simulink model "case2"  (R2024b)
settings: Solver=FixedStepAuto  StartTime=0  StopTime=1  FixedStep=1e-7  RelTol=1e-3
values from neighbouring files (symbols this model uses):
  SG_D_1_D = 0.01056    [IEEE9_case_parameters.m]    (also in case1_parameters.m; case2_parameters.m; case3_parameters.m; case4_parameters.m)
  SG_D_1_EnableSaturation = 0    [IEEE9_case_parameters.m]    (also in case1_parameters.m; case2_parameters.m; case3_parameters.m; case4_parameters.m)
  SG_D_1_f0 = 60    [IEEE9_case_parameters.m]    (also in case1_parameters.m; case2_parameters.m; case3_parameters.m; case4_parameters.m)
  SG_D_1_H = 7.5    [IEEE9_case_parameters.m]    (also in case1_parameters.m; case2_parameters.m; case3_parameters.m; case4_parameters.m)
  SG_D_1_K_A = 20    [IEEE9_case_parameters.m]    (also in case1_parameters.m; case2_parameters.m; case3_parameters.m; case4_parameters.m)
  SG_D_1_K_E = 1.000000e+1    (= 10)    [IEEE9_case_parameters.m]    (also in case1_parameters.m; case2_parameters.m; case3_parameters.m; case4_parameters.m)
  SG_D_1_K_F = 2.363    [IEEE9_case_parameters.m]    (also in case1_parameters.m; case2_parameters.m; case3_parameters.m; case4_parameters.m)
  SG_D_1_K_s = 0.5    [IEEE9_case_parameters.m]    (also in case1_parameters.m = 5; case2_parameters.m = 5; case3_parameters.m = 5; case4_parameters.m = 5)
  SG_D_1_R_a = 0.001088    [IEEE9_case_parameters.m]    (also in case1_parameters.m; case2_parameters.m; case3_parameters.m; case4_parameters.m)
  SG_D_1_S_A = 1    [IEEE9_case_parameters.m]    (also in case1_parameters.m; case2_parameters.m; case3_parameters.m; case4_parameters.m)
  SG_D_1_S_B = 0.103    [IEEE9_case_parameters.m]    (also in case1_parameters.m; case2_parameters.m; case3_parameters.m; case4_parameters.m)
  SG_D_1_S_N = 10.659857    [IEEE9_case_parameters.m]    (also in case1_parameters.m; case2_parameters.m; case3_parameters.m; case4_parameters.m)
  SG_D_1_SpeedPara = 200    [IEEE9_case_parameters.m]    (also in case1_parameters.m; case2_parameters.m; case3_parameters.m; case4_parameters.m)
  SG_D_1_T_0 = 0.720173    [IEEE9_case_parameters.m]    (also in case1_parameters.m = 0.755522; case2_parameters.m = 0.808931; case3_parameters.m = 0.869402; case4_parameters.m = 0.729316)
  SG_D_1_T_1 = 0.3    [IEEE9_case_parameters.m]    (also in case1_parameters.m; case2_parameters.m; case3_parameters.m; case4_parameters.m)
  SG_D_1_T_2 = 0.05    [IEEE9_case_parameters.m]    (also in case1_parameters.m; case2_parameters.m; case3_parameters.m; case4_parameters.m)
  SG_D_1_T_3 = 0.02    [IEEE9_case_parameters.m]    (also in case1_parameters.m; case2_parameters.m; case3_parameters.m; case4_parameters.m)
  SG_D_1_T_4 = 0.005    [IEEE9_case_parameters.m]    (also in case1_parameters.m; case2_parameters.m; case3_parameters.m; case4_parameters.m)
  SG_D_1_T_A = 0.02    [IEEE9_case_parameters.m]    (also in case1_parameters.m; case2_parameters.m; case3_parameters.m; case4_parameters.m)
  SG_D_1_T_dd = 8.000000e+0    (= 8)    [IEEE9_case_parameters.m]    (also in case1_parameters.m; case2_parameters.m; case3_parameters.m; case4_parameters.m)
  SG_D_1_T_ddd = 0.04    [IEEE9_case_parameters.m]    (also in case1_parameters.m; case2_parameters.m; case3_parameters.m; case4_parameters.m)
  SG_D_1_T_E = 0.314    [IEEE9_case_parameters.m]    (also in case1_parameters.m; case2_parameters.m; case3_parameters.m; case4_parameters.m)
  SG_D_1_T_F = 0.35    [IEEE9_case_parameters.m]    (also in case1_parameters.m; case2_parameters.m; case3_parameters.m; case4_parameters.m)
  SG_D_1_T_qd = 0.8    [IEEE9_case_parameters.m]    (also in case1_parameters.m; case2_parameters.m; case3_parameters.m; case4_parameters.m)
  SG_D_1_T_qdd = 0.02    [IEEE9_case_parameters.m]    (also in case1_parameters.m; case2_parameters.m; case3_parameters.m; case4_parameters.m)
  SG_D_1_T_speed = 0.1    [IEEE9_case_parameters.m]    (also in case1_parameters.m = 200; case2_parameters.m = 200; case3_parameters.m = 200; case4_parameters.m = 200)
  SG_D_1_T_w = 0.5    [IEEE9_case_parameters.m]    (also in case1_parameters.m; case2_parameters.m; case3_parameters.m; case4_parameters.m)
  SG_D_1_V_ref = 1.990276    [IEEE9_case_parameters.m]    (also in case1_parameters.m = 2.042296; case2_parameters.m = 2.051388; case3_parameters.m = 2.089584; case4_parameters.m = 2.01845)
  SG_D_1_w_ref = 376.991118    [IEEE9_case_parameters.m]    (also in case1_parameters.m; case2_parameters.m; case3_parameters.m; case4_parameters.m)
  SG_D_1_wb = 6.000000e+1    (= 60)    [IEEE9_case_parameters.m]    (also in case1_parameters.m; case2_parameters.m; case3_parameters.m; case4_parameters.m)
  SG_D_1_x_d = 1.9    [IEEE9_case_parameters.m]    (also in case1_parameters.m; case2_parameters.m; case3_parameters.m; case4_parameters.m)
  SG_D_1_x_dd = 0.302    [IEEE9_case_parameters.m]    (also in case1_parameters.m; case2_parameters.m; case3_parameters.m; case4_parameters.m)
  SG_D_1_x_ddd = 0.204    [IEEE9_case_parameters.m]    (also in case1_parameters.m; case2_parameters.m; case3_parameters.m; case4_parameters.m)
  SG_D_1_x_l = 0.05    [IEEE9_case_parameters.m]    (also in case1_parameters.m; case2_parameters.m; case3_parameters.m; case4_parameters.m)
  SG_D_1_x_q = 1.3    [IEEE9_case_parameters.m]    (also in case1_parameters.m; case2_parameters.m; case3_parameters.m; case4_parameters.m)
  SG_D_1_x_qd = 0.5    [IEEE9_case_parameters.m]    (also in case1_parameters.m; case2_parameters.m; case3_parameters.m; case4_parameters.m)
  SG_D_1_x_qdd = 0.3    [IEEE9_case_parameters.m]    (also in case1_parameters.m; case2_parameters.m; case3_parameters.m; case4_parameters.m)
  SG_D_2_D = 0.02    [IEEE9_case_parameters.m]    (also in case1_parameters.m; case2_parameters.m; case3_parameters.m; case4_parameters.m)
  SG_D_2_EnableSaturation = 0    [IEEE9_case_parameters.m]    (also in case1_parameters.m; case2_parameters.m; case3_parameters.m; case4_parameters.m)
  SG_D_2_f0 = 60    [IEEE9_case_parameters.m]    (also in case1_parameters.m; case2_parameters.m; case3_parameters.m; case4_parameters.m)
  SG_D_2_H = 8.000000e+0    (= 8)    [IEEE9_case_parameters.m]    (also in case1_parameters.m; case2_parameters.m; case3_parameters.m; case4_parameters.m)
  SG_D_2_K_A = 20    [IEEE9_case_parameters.m]    (also in case1_parameters.m; case2_parameters.m; case3_parameters.m; case4_parameters.m)
  SG_D_2_K_E = 1.000000e+1    (= 10)    [IEEE9_case_parameters.m]    (also in case1_parameters.m; case2_parameters.m; case3_parameters.m; case4_parameters.m)
  SG_D_2_K_F = 2.363    [IEEE9_case_parameters.m]    (also in case1_parameters.m; case2_parameters.m; case3_parameters.m; case4_parameters.m)
  SG_D_2_K_s = 0.5    [IEEE9_case_parameters.m]    (also in case1_parameters.m = 4; case2_parameters.m = 4; case3_parameters.m = 4; case4_parameters.m = 4)
  SG_D_2_R_a = 0.001088    [IEEE9_case_parameters.m]    (also in case1_parameters.m; case2_parameters.m; case3_parameters.m; case4_parameters.m)
  SG_D_2_S_A = 1    [IEEE9_case_parameters.m]    (also in case1_parameters.m; case2_parameters.m; case3_parameters.m; case4_parameters.m)
  SG_D_2_S_B = 0.103    [IEEE9_case_parameters.m]    (also in case1_parameters.m; case2_parameters.m; case3_parameters.m; case4_parameters.m)
  SG_D_2_S_N = 10.659857    [IEEE9_case_parameters.m]    (also in case1_parameters.m; case2_parameters.m; case3_parameters.m; case4_parameters.m)
  SG_D_2_SpeedPara = 200    [IEEE9_case_parameters.m]    (also in case1_parameters.m; case2_parameters.m; case3_parameters.m; case4_parameters.m)
  SG_D_2_T_0 = 1.632913    [IEEE9_case_parameters.m]    (also in case1_parameters.m = 1.632925; case2_parameters.m = 1.632915; case3_parameters.m = 1.632914; case4_parameters.m = 1.632927)
  SG_D_2_T_1 = 0.2    [IEEE9_case_parameters.m]    (also in case1_parameters.m; case2_parameters.m; case3_parameters.m; case4_parameters.m)
  SG_D_2_T_2 = 0.05    [IEEE9_case_parameters.m]    (also in case1_parameters.m; case2_parameters.m; case3_parameters.m; case4_parameters.m)
  SG_D_2_T_3 = 0.02    [IEEE9_case_parameters.m]    (also in case1_parameters.m; case2_parameters.m; case3_parameters.m; case4_parameters.m)
  SG_D_2_T_4 = 0.005    [IEEE9_case_parameters.m]    (also in case1_parameters.m; case2_parameters.m; case3_parameters.m; case4_parameters.m)
  SG_D_2_T_A = 0.02    [IEEE9_case_parameters.m]    (also in case1_parameters.m; case2_parameters.m; case3_parameters.m; case4_parameters.m)
  SG_D_2_T_dd = 7.9    [IEEE9_case_parameters.m]    (also in case1_parameters.m; case2_parameters.m; case3_parameters.m; case4_parameters.m)
  SG_D_2_T_ddd = 0.04    [IEEE9_case_parameters.m]    (also in case1_parameters.m; case2_parameters.m; case3_parameters.m; case4_parameters.m)
  SG_D_2_T_E = 0.314    [IEEE9_case_parameters.m]    (also in case1_parameters.m; case2_parameters.m; case3_parameters.m; case4_parameters.m)
  SG_D_2_T_F = 0.35    [IEEE9_case_parameters.m]    (also in case1_parameters.m; case2_parameters.m; case3_parameters.m; case4_parameters.m)
  SG_D_2_T_qd = 0.8    [IEEE9_case_parameters.m]    (also in case1_parameters.m; case2_parameters.m; case3_parameters.m; case4_parameters.m)
  SG_D_2_T_qdd = 0.015    [IEEE9_case_parameters.m]    (also in case1_parameters.m; case2_parameters.m; case3_parameters.m; case4_parameters.m)
  SG_D_2_T_speed = 0.1    [IEEE9_case_parameters.m]    (also in case1_parameters.m = 150; case2_parameters.m = 150; case3_parameters.m = 150; case4_parameters.m = 150)
  SG_D_2_T_w = 0.35    [IEEE9_case_parameters.m]    (also in case1_parameters.m; case2_parameters.m; case3_parameters.m; case4_parameters.m)
  SG_D_2_V_ref = 2.58547    [IEEE9_case_parameters.m]    (also in case1_parameters.m = 2.597896; case2_parameters.m = 2.587136; case3_parameters.m = 2.586042; case4_parameters.m = 2.599679)
  SG_D_2_w_ref = 376.991118    [IEEE9_case_parameters.m]    (also in case1_parameters.m; case2_parameters.m; case3_parameters.m; case4_parameters.m)
  SG_D_2_wb = 6.000000e+1    (= 60)    [IEEE9_case_parameters.m]    (also in case1_parameters.m; case2_parameters.m; case3_parameters.m; case4_parameters.m)
  SG_D_2_x_d = 1.8    [IEEE9_case_parameters.m]    (also in case1_parameters.m; case2_parameters.m; case3_parameters.m; case4_parameters.m)
  SG_D_2_x_dd = 0.302    [IEEE9_case_parameters.m]    (also in case1_parameters.m; case2_parameters.m; case3_parameters.m; case4_parameters.m)
  SG_D_2_x_ddd = 0.204    [IEEE9_case_parameters.m]    (also in case1_parameters.m; case2_parameters.m; case3_parameters.m; case4_parameters.m)
  SG_D_2_x_l = 0.05    [IEEE9_case_parameters.m]    (also in case1_parameters.m; case2_parameters.m; case3_parameters.m; case4_parameters.m)
  SG_D_2_x_q = 1.25    [IEEE9_case_parameters.m]    (also in case1_parameters.m; case2_parameters.m; case3_parameters.m; case4_parameters.m)
  SG_D_2_x_qd = 0.5    [IEEE9_case_parameters.m]    (also in case1_parameters.m; case2_parameters.m; case3_parameters.m; case4_parameters.m)
  SG_D_2_x_qdd = 0.3    [IEEE9_case_parameters.m]    (also in case1_parameters.m; case2_parameters.m; case3_parameters.m; case4_parameters.m)
  SG_D_3_D = 0.02    [IEEE9_case_parameters.m]    (also in case1_parameters.m; case2_parameters.m; case3_parameters.m; case4_parameters.m)
  SG_D_3_EnableSaturation = 0    [IEEE9_case_parameters.m]    (also in case1_parameters.m; case2_parameters.m; case3_parameters.m; case4_parameters.m)
  SG_D_3_f0 = 60    [IEEE9_case_parameters.m]    (also in case1_parameters.m; case2_parameters.m; case3_parameters.m; case4_parameters.m)
  SG_D_3_H = 7.7    [IEEE9_case_parameters.m]    (also in case1_parameters.m; case2_parameters.m; case3_parameters.m; case4_parameters.m)
  SG_D_3_K_A = 20    [IEEE9_case_parameters.m]    (also in case1_parameters.m; case2_parameters.m; case3_parameters.m; case4_parameters.m)
  SG_D_3_K_E = 1.000000e+1    (= 10)    [IEEE9_case_parameters.m]    (also in case1_parameters.m; case2_parameters.m; case3_parameters.m; case4_parameters.m)
  SG_D_3_K_F = 2.363    [IEEE9_case_parameters.m]    (also in case1_parameters.m; case2_parameters.m; case3_parameters.m; case4_parameters.m)
  SG_D_3_K_s = 0.2    [IEEE9_case_parameters.m]    (also in case1_parameters.m = 2; case2_parameters.m = 2; case3_parameters.m = 2; case4_parameters.m = 2)
  SG_D_3_R_a = 0.001088    [IEEE9_case_parameters.m]    (also in case1_parameters.m; case2_parameters.m; case3_parameters.m; case4_parameters.m)
  SG_D_3_S_A = 1    [IEEE9_case_parameters.m]    (also in case1_parameters.m; case2_parameters.m; case3_parameters.m; case4_parameters.m)
  SG_D_3_S_B = 0.103    [IEEE9_case_parameters.m]    (also in case1_parameters.m; case2_parameters.m; case3_parameters.m; case4_parameters.m)
  SG_D_3_S_N = 10.659857    [IEEE9_case_parameters.m]    (also in case1_parameters.m; case2_parameters.m; case3_parameters.m; case4_parameters.m)
  SG_D_3_SpeedPara = 200    [IEEE9_case_parameters.m]    (also in case1_parameters.m; case2_parameters.m; case3_parameters.m; case4_parameters.m)
  SG_D_3_T_0 = 0.850788    [IEEE9_case_parameters.m]    (also in case1_parameters.m = 0.850786; case2_parameters.m = 0.850787; case3_parameters.m; case4_parameters.m = 0.850786)
  SG_D_3_T_1 = 0.2    [IEEE9_case_parameters.m]    (also in case1_parameters.m; case2_parameters.m; case3_parameters.m; case4_parameters.m)
  SG_D_3_T_2 = 0.05    [IEEE9_case_parameters.m]    (also in case1_parameters.m; case2_parameters.m; case3_parameters.m; case4_parameters.m)
  SG_D_3_T_3 = 0.02    [IEEE9_case_parameters.m]    (also in case1_parameters.m; case2_parameters.m; case3_parameters.m; case4_parameters.m)
  SG_D_3_T_4 = 0.005    [IEEE9_case_parameters.m]    (also in case1_parameters.m; case2_parameters.m; case3_parameters.m; case4_parameters.m)
  SG_D_3_T_A = 0.02    [IEEE9_case_parameters.m]    (also in case1_parameters.m; case2_parameters.m; case3_parameters.m; case4_parameters.m)
  SG_D_3_T_dd = 8.1    [IEEE9_case_parameters.m]    (also in case1_parameters.m; case2_parameters.m; case3_parameters.m; case4_parameters.m)
  SG_D_3_T_ddd = 0.04    [IEEE9_case_parameters.m]    (also in case1_parameters.m; case2_parameters.m; case3_parameters.m; case4_parameters.m)
  SG_D_3_T_E = 0.314    [IEEE9_case_parameters.m]    (also in case1_parameters.m; case2_parameters.m; case3_parameters.m; case4_parameters.m)
  SG_D_3_T_F = 0.35    [IEEE9_case_parameters.m]    (also in case1_parameters.m; case2_parameters.m; case3_parameters.m; case4_parameters.m)
  SG_D_3_T_qd = 0.8    [IEEE9_case_parameters.m]    (also in case1_parameters.m; case2_parameters.m; case3_parameters.m; case4_parameters.m)
  SG_D_3_T_qdd = 0.015    [IEEE9_case_parameters.m]    (also in case1_parameters.m; case2_parameters.m; case3_parameters.m; case4_parameters.m)
  SG_D_3_T_speed = 0.1    [IEEE9_case_parameters.m]    (also in case1_parameters.m = 180; case2_parameters.m = 180; case3_parameters.m = 180; case4_parameters.m = 180)
  SG_D_3_T_w = 0.4    [IEEE9_case_parameters.m]    (also in case1_parameters.m; case2_parameters.m; case3_parameters.m; case4_parameters.m)
  SG_D_3_V_ref = 1.892727    [IEEE9_case_parameters.m]    (also in case1_parameters.m = 1.906439; case2_parameters.m = 1.895535; case3_parameters.m = 1.892105; case4_parameters.m = 1.906598)
  SG_D_3_w_ref = 376.991118    [IEEE9_case_parameters.m]    (also in case1_parameters.m; case2_parameters.m; case3_parameters.m; case4_parameters.m)
  SG_D_3_wb = 6.000000e+1    (= 60)    [IEEE9_case_parameters.m]    (also in case1_parameters.m; case2_parameters.m; case3_parameters.m; case4_parameters.m)
  SG_D_3_x_d = 1.85    [IEEE9_case_parameters.m]    (also in case1_parameters.m; case2_parameters.m; case3_parameters.m; case4_parameters.m)
  SG_D_3_x_dd = 0.302    [IEEE9_case_parameters.m]    (also in case1_parameters.m; case2_parameters.m; case3_parameters.m; case4_parameters.m)
  SG_D_3_x_ddd = 0.204    [IEEE9_case_parameters.m]    (also in case1_parameters.m; case2_parameters.m; case3_parameters.m; case4_parameters.m)
  SG_D_3_x_l = 0.05    [IEEE9_case_parameters.m]    (also in case1_parameters.m; case2_parameters.m; case3_parameters.m; case4_parameters.m)
  SG_D_3_x_q = 1.2    [IEEE9_case_parameters.m]    (also in case1_parameters.m; case2_parameters.m; case3_parameters.m; case4_parameters.m)
  SG_D_3_x_qd = 0.5    [IEEE9_case_parameters.m]    (also in case1_parameters.m; case2_parameters.m; case3_parameters.m; case4_parameters.m)
  SG_D_3_x_qdd = 0.3    [IEEE9_case_parameters.m]    (also in case1_parameters.m; case2_parameters.m; case3_parameters.m; case4_parameters.m)
(part 5 of 12)

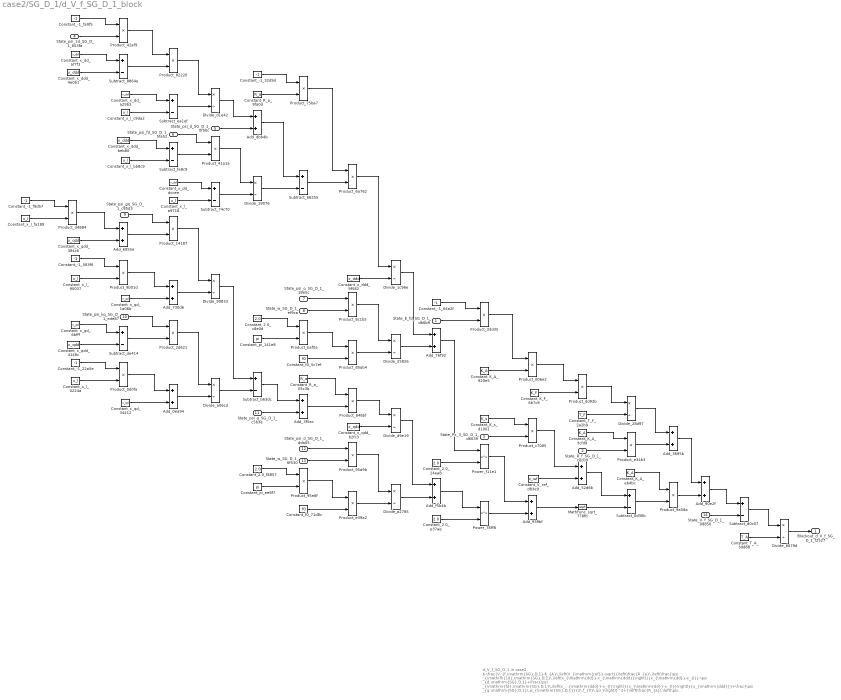
== system case2/SG_D_1/d_V_f_SG_D_1_block ==
  note: d_V_f_SG_D_1 in case2
      | $-\frac{V_{f,\mathrm{SG},D,1}-K_{A}\,\left(V_{\mathrm{ref}}-\sqrt{{\left(\frac{R_{a}\,\left(\frac{\psi _{\mathrm{1d},\mathrm{SG},D,1}\,\left(x_{\mathrm{dd}}-x_{\mathrm{ddd}}\right)}{x_{\mathrm{dd}}-x_{l}}-\psi _{d,\mathrm{SG},D,1}+\frac{\psi _{\mathrm{fd},\mathrm{SG},D,1}\,\left(x_{\mathrm{ddd}}-x_{l}\right)}{x_{\mathrm{dd}}-x_{l}}\right)}{x_{\mathrm{ddd}}}+\frac{\psi _{q,\mathrm{SG},D,1}\,w_{\mathrm{SG},D,1}}{2\,f_{0}\,\pi }\right)}^2+{\left(\frac{R_{a}\,\left(\psi _{q,\mathrm{SG},D,1}+\frac{\psi _{\mathrm{gq},\mathrm{SG},D,1}\,\left(x_{l}-x_{\mathrm{qdd}}\right)}{x_{l}-x_{\mathrm{qd}}}+\frac{\psi _{\mathrm{kq},\mathrm{SG},D,1}\,\left(x_{\mathrm{qd}}-x_{\mathrm{qdd}}\right)}{x_{l}-x_{\mathrm{qd}}}\right)}{x_{\mathrm{qdd}}}+\frac{\psi _{d,\mathrm{SG},D,1}\,w_{\mathrm{SG},D,1}}{2\,f_{0}\,\pi }\right)}^2}+K_{s}\,\mathrm{Px}_{3,\mathrm{SG},D,1}\right)-K_{A}\,R_{f,\mathrm{SG},D,1}+\frac{E_{\mathrm{fd},\mathrm{SG},D,1}\,K_{A}\,K_{F}}{T_{F}}}{T_{A}}$
      | Automatically generated on 2025-10-31 18:53:39 .
  State_E_fd_SG_D_1_db6b9 : Inport
  State_R_f_SG_D_1_cec09 : Inport  Port=2
  State_Px_3_SG_D_1_d6039 : Inport  Port=3
  State_psi_1d_SG_D_1_653fa : Inport  Port=4
  State_psi_d_SG_D_1_0f50c : Inport  Port=5
  State_psi_fd_SG_D_1_5fa52 : Inport  Port=6
  State_psi_q_SG_D_1_18e5c : Inport  Port=7
  State_w_SG_D_1_ef9ca : Inport  Port=8
  State_psi_gq_SG_D_1_c85d3 : Inport  Port=9
  State_psi_kq_SG_D_1_ede87 : Inport  Port=10
  State_psi_q_SG_D_1_c5b3e : Inport  Port=11
  State_psi_d_SG_D_1_dda05 : Inport  Port=12
  State_w_SG_D_1_6f530 : Inport  Port=13
  State_V_f_SG_D_1_0d850 : Inport  Port=14
  Add_0ea94 : Sum
  Add_3695b : Sum
  Add_3f5ac : Sum
  Add_52d6b : Sum
  Add_6955e : Sum
  Add_730d6 : Sum
  Add_76f92 : Sum
  Add_90e2f : Sum
  Add_939bf : Sum
  Add_dbb4b : Sum
  Add_f5b4b : Sum
  Constant_-1_22a5e : Constant  Value=-1
  Constant_-1_32d9d : Constant  Value=-1
  Constant_-1_583f6 : Constant  Value=-1
  Constant_-1_64a2f : Constant  Value=-1
  Constant_-1_f9d57 : Constant  Value=-1
  Constant_-1_fa9f5 : Constant  Value=-1
  Constant_2.0_24ea8 : Constant  Value=2.0
  Constant_2.0_c8e0d : Constant  Value=2.0
  Constant_2.0_e37ae : Constant  Value=2.0
  Constant_2.0_f8857 : Constant  Value=2.0
  Constant_K_A_3cfd9 : Constant  Value=K_A
  Constant_K_A_920e5 : Constant  Value=K_A
  Constant_K_A_eb4bc : Constant  Value=K_A
  Constant_K_F_6b7c9 : Constant  Value=K_F
  Constant_K_s_d1001 : Constant  Value=K_s
  Constant_R_a_05c3b : Constant  Value=R_a
  Constant_R_a_9fa0d : Constant  Value=R_a
  Constant_T_A_3dd88 : Constant  Value=T_A
  Constant_T_F_2a2b9 : Constant  Value=T_F
  Constant_V_ref_d83e9 : Constant  Value=V_ref
  Constant_f0_5c7ef : Constant  Value=f0
  Constant_f0_71d8c : Constant  Value=f0
  Constant_pi_141e8 : Constant  Value=pi
  Constant_pi_ee8f7 : Constant  Value=pi
  Constant_x_dd_a29b3 : Constant  Value=x_dd
  Constant_x_dd_af7f3 : Constant  Value=x_dd
  Constant_x_dd_dccee : Constant  Value=x_dd
  Constant_x_ddd_4e0b1 : Constant  Value=x_ddd
  Constant_x_ddd_9f582 : Constant  Value=x_ddd
  Constant_x_ddd_beb80 : Constant  Value=x_ddd
  Constant_x_l_0224a : Constant  Value=x_l
  Constant_x_l_90037 : Constant  Value=x_l
  Constant_x_l_a9718 : Constant  Value=x_l
  Constant_x_l_bb8c9 : Constant  Value=x_l
  Constant_x_l_c9da2 : Constant  Value=x_l
  Constant_x_l_fa189 : Constant  Value=x_l
  Constant_x_qd_1a06b : Constant  Value=x_qd
  Constant_x_qd_34412 : Constant  Value=x_qd
  Constant_x_qd_6bfff : Constant  Value=x_qd
  Constant_x_qdd_384c6 : Constant  Value=x_qdd
  Constant_x_qdd_4148c : Constant  Value=x_qdd
  Constant_x_qdd_b2fc3 : Constant  Value=x_qdd
  Divide_19076 : Product  Inputs=*/
  Divide_1c96e : Product  Inputs=*/
  Divide_25826 : Product  Inputs=*/
  Divide_28d97 : Product  Inputs=*/
  Divide_6679d : Product  Inputs=*/
  Divide_90833 : Product  Inputs=*/
  Divide_a06cd : Product  Inputs=*/
  Divide_a2785 : Product  Inputs=*/
  Divide_d1e42 : Product  Inputs=*/
  Divide_d9e19 : Product  Inputs=*/
  MathFunc_sqrt_778fb : Sqrt
  Power_35ff8 : Math  Operator=pow
  Power_f11e1 : Math  Operator=pow
  Product_006e2 : Product
  Product_0d0fa : Product
  Product_14187 : Product
  Product_2d621 : Product
  Product_33d35 : Product
  Product_41a1a : Product
  Product_42af9 : Product
  Product_6a762 : Product
  Product_75ba7 : Product
  Product_82220 : Product
  Product_848bf : Product
  Product_85ab4 : Product
  Product_8c1b5 : Product
  Product_95a9b : Product
  Product_95e8f : Product
  Product_9a58a : Product
  Product_9b01d : Product
  Product_baf0a : Product
  Product_c7085 : Product
  Product_d4884 : Product
  Product_dd92b : Product
  Product_e34b3 : Product
  Product_e39a2 : Product
  Subtract_0d36b : Sum  Inputs=+-
  Subtract_66255 : Sum  Inputs=+-
  Subtract_74c70 : Sum  Inputs=+-
  Subtract_8864e : Sum  Inputs=+-
  Subtract_b63dc : Sum  Inputs=+-
  Subtract_d0c07 : Sum  Inputs=+-
  Subtract_de414 : Sum  Inputs=+-
  Subtract_ea1ef : Sum  Inputs=+-
  Subtract_fa8c9 : Sum  Inputs=+-
  Blockout_d_V_f_SG_D_1_f2527 : Outport
  wires:
  Constant_-1_22a5e/1 -> Product_0d0fa/1
  Constant_-1_f9d57/1 -> Product_d4884/1
  State_psi_d_SG_D_1_dda05/1 -> Product_95a9b/1
  Constant_x_qd_34412/1 -> Add_0ea94/2
  Constant_x_qdd_384c6/1 -> Add_6955e/2
  State_w_SG_D_1_6f530/1 -> Product_95a9b/2
  Constant_x_l_fa189/1 -> Product_d4884/2
  Subtract_66255/1 -> Product_6a762/2
  Constant_x_l_0224a/1 -> Product_0d0fa/2
  Constant_x_dd_af7f3/1 -> Subtract_8864e/1
  Constant_R_a_9fa0d/1 -> Product_75ba7/2
  Constant_-1_fa9f5/1 -> Product_42af9/1
  Divide_19076/1 -> Subtract_66255/2
  Constant_x_ddd_4e0b1/1 -> Subtract_8864e/2
  Add_0ea94/1 -> Divide_a06cd/2
  State_psi_1d_SG_D_1_653fa/1 -> Product_42af9/2
  Add_730d6/1 -> Divide_90833/2
  Subtract_de414/1 -> Product_2d621/2
  Product_dd92b/1 -> Divide_28d97/1
  Product_baf0a/1 -> Product_85ab4/1
  Product_d4884/1 -> Add_6955e/1
  Constant_-1_583f6/1 -> Product_9b01d/1
  Constant_x_l_90037/1 -> Product_9b01d/2
  Add_dbb4b/1 -> Subtract_66255/1
  Constant_2.0_f8857/1 -> Product_95e8f/1
  Constant_x_qd_6bfff/1 -> Subtract_de414/1
  Product_42af9/1 -> Product_82220/1
  Constant_pi_ee8f7/1 -> Product_95e8f/2
  Constant_x_qdd_4148c/1 -> Subtract_de414/2
  Subtract_8864e/1 -> Product_82220/2
  State_psi_q_SG_D_1_c5b3e/1 -> Add_3f5ac/2
  Constant_x_dd_a29b3/1 -> Subtract_ea1ef/1
  Constant_x_l_c9da2/1 -> Subtract_ea1ef/2
  Constant_x_ddd_beb80/1 -> Subtract_fa8c9/1
  Constant_x_l_bb8c9/1 -> Subtract_fa8c9/2
  State_psi_gq_SG_D_1_c85d3/1 -> Product_14187/1
  Add_6955e/1 -> Product_14187/2
  Product_9b01d/1 -> Add_730d6/1
  Constant_x_qd_1a06b/1 -> Add_730d6/2
  Divide_d1e42/1 -> Add_dbb4b/1
  Subtract_ea1ef/1 -> Divide_d1e42/2
  State_psi_kq_SG_D_1_ede87/1 -> Product_2d621/1
  Divide_6679d/1 -> Blockout_d_V_f_SG_D_1_f2527/1
  Product_0d0fa/1 -> Add_0ea94/1
  Product_82220/1 -> Divide_d1e42/1
  State_psi_fd_SG_D_1_5fa52/1 -> Product_41a1a/1
  State_w_SG_D_1_ef9ca/1 -> Product_8c1b5/2
  Subtract_fa8c9/1 -> Product_41a1a/2
  Constant_x_dd_dccee/1 -> Subtract_74c70/1
  Constant_x_l_a9718/1 -> Subtract_74c70/2
  Product_14187/1 -> Divide_90833/1
  Product_75ba7/1 -> Product_6a762/1
  Product_2d621/1 -> Divide_a06cd/1
  State_psi_d_SG_D_1_0f50c/1 -> Add_dbb4b/2
  Product_41a1a/1 -> Divide_19076/1
  Subtract_74c70/1 -> Divide_19076/2
  Divide_90833/1 -> Subtract_b63dc/1
  Divide_a06cd/1 -> Subtract_b63dc/2
  Constant_-1_32d9d/1 -> Product_75ba7/1
  Constant_2.0_c8e0d/1 -> Product_baf0a/1
  Constant_pi_141e8/1 -> Product_baf0a/2
  Subtract_b63dc/1 -> Add_3f5ac/1
  State_psi_q_SG_D_1_18e5c/1 -> Product_8c1b5/1
  Constant_f0_5c7ef/1 -> Product_85ab4/2
  Constant_R_a_05c3b/1 -> Product_848bf/1
  Add_3f5ac/1 -> Product_848bf/2
  Product_95e8f/1 -> Product_e39a2/1
  Power_f11e1/1 -> Add_939bf/1
  Constant_f0_71d8c/1 -> Product_e39a2/2
  Product_6a762/1 -> Divide_1c96e/1
  Constant_x_ddd_9f582/1 -> Divide_1c96e/2
  Product_8c1b5/1 -> Divide_25826/1
  Product_85ab4/1 -> Divide_25826/2
  Product_848bf/1 -> Divide_d9e19/1
  Constant_x_qdd_b2fc3/1 -> Divide_d9e19/2
  Product_95a9b/1 -> Divide_a2785/1
  Product_e39a2/1 -> Divide_a2785/2
  Divide_1c96e/1 -> Add_76f92/1
  Divide_25826/1 -> Add_76f92/2
  Divide_d9e19/1 -> Add_f5b4b/1
  Divide_a2785/1 -> Add_f5b4b/2
  Constant_-1_64a2f/1 -> Product_33d35/1
  State_E_fd_SG_D_1_db6b9/1 -> Product_33d35/2
  Add_76f92/1 -> Power_f11e1/1
  Constant_2.0_24ea8/1 -> Power_f11e1/2
  Add_f5b4b/1 -> Power_35ff8/1
  Constant_2.0_e37ae/1 -> Power_35ff8/2
  Product_33d35/1 -> Product_006e2/1
  Constant_K_A_920e5/1 -> Product_006e2/2
  Constant_K_s_d1001/1 -> Product_c7085/1
  State_Px_3_SG_D_1_d6039/1 -> Product_c7085/2
  Power_35ff8/1 -> Add_939bf/2
  Divide_28d97/1 -> Add_3695b/1
  Product_006e2/1 -> Product_dd92b/1
  Constant_K_F_6b7c9/1 -> Product_dd92b/2
  Product_c7085/1 -> Add_52d6b/1
  Constant_V_ref_d83e9/1 -> Add_52d6b/2
  Add_939bf/1 -> MathFunc_sqrt_778fb/1
  Constant_T_F_2a2b9/1 -> Divide_28d97/2
  Constant_K_A_3cfd9/1 -> Product_e34b3/1
  State_R_f_SG_D_1_cec09/1 -> Product_e34b3/2
  Add_52d6b/1 -> Subtract_0d36b/1
  MathFunc_sqrt_778fb/1 -> Subtract_0d36b/2
  Constant_T_A_3dd88/1 -> Divide_6679d/2
  Product_e34b3/1 -> Add_3695b/2
  Constant_K_A_eb4bc/1 -> Product_9a58a/1
  Subtract_0d36b/1 -> Product_9a58a/2
  Add_3695b/1 -> Add_90e2f/1
  Product_9a58a/1 -> Add_90e2f/2
  Add_90e2f/1 -> Subtract_d0c07/1
  State_V_f_SG_D_1_0d850/1 -> Subtract_d0c07/2
  Subtract_d0c07/1 -> Divide_6679d/1

== system case2/SG_D_1/d_psi_1d_SG_D_1_block ==
  note: d_psi_1d_SG_D_1 in case2
      | $-\frac{\psi _{\mathrm{1d},\mathrm{SG},D,1}-\psi _{\mathrm{fd},\mathrm{SG},D,1}+\frac{\left(x_{\mathrm{dd}}-x_{l}\right)\,\left(\frac{\psi _{\mathrm{1d},\mathrm{SG},D,1}\,\left(x_{\mathrm{dd}}-x_{\mathrm{ddd}}\right)}{x_{\mathrm{dd}}-x_{l}}-\psi _{d,\mathrm{SG},D,1}+\frac{\psi _{\mathrm{fd},\mathrm{SG},D,1}\,\left(x_{\mathrm{ddd}}-x_{l}\right)}{x_{\mathrm{dd}}-x_{l}}\right)}{x_{\mathrm{ddd}}}}{T_{\mathrm{ddd}}}$
      | Automatically generated on 2025-10-31 18:53:13 .
  State_psi_1d_SG_D_1_9b7db : Inport
  State_psi_fd_SG_D_1_cc7fa : Inport  Port=2
  State_psi_1d_SG_D_1_c2340 : Inport  Port=3
  State_psi_d_SG_D_1_fa460 : Inport  Port=4
  State_psi_fd_SG_D_1_43baf : Inport  Port=5
  Add_85150 : Sum
  Add_8d5e1 : Sum
  Add_e7ea3 : Sum
  Constant_-1_4ea77 : Constant  Value=-1
  Constant_-1_96109 : Constant  Value=-1
  Constant_T_ddd_e98c2 : Constant  Value=T_ddd
  Constant_x_dd_3736a : Constant  Value=x_dd
  Constant_x_dd_aeb06 : Constant  Value=x_dd
  Constant_x_dd_c7d7e : Constant  Value=x_dd
  Constant_x_dd_c88ae : Constant  Value=x_dd
  Constant_x_ddd_23f75 : Constant  Value=x_ddd
  Constant_x_ddd_7d76a : Constant  Value=x_ddd
  Constant_x_ddd_b9df0 : Constant  Value=x_ddd
  Constant_x_l_14475 : Constant  Value=x_l
  Constant_x_l_8dddb : Constant  Value=x_l
  Constant_x_l_e512f : Constant  Value=x_l
  Constant_x_l_f444c : Constant  Value=x_l
  Divide_50057 : Product  Inputs=*/
  Divide_91c72 : Product  Inputs=*/
  Divide_9ad1a : Product  Inputs=*/
  Divide_b306c : Product  Inputs=*/
  Product_46e69 : Product
  Product_89b52 : Product
  Product_a7042 : Product
  Product_ce9a5 : Product
  Product_f0574 : Product
  Subtract_1b8e7 : Sum  Inputs=+-
  Subtract_21993 : Sum  Inputs=+-
  Subtract_aa06c : Sum  Inputs=+-
  Subtract_aa658 : Sum  Inputs=+-
  Subtract_b850d : Sum  Inputs=+-
  Subtract_d68dd : Sum  Inputs=+-
  Blockout_d_psi_1d_SG_D_1_2ff74 : Outport
  wires:
  Product_ce9a5/1 -> Product_46e69/1
  Constant_-1_4ea77/1 -> Product_ce9a5/1
  Subtract_d68dd/1 -> Product_46e69/2
  State_psi_1d_SG_D_1_c2340/1 -> Product_ce9a5/2
  Subtract_1b8e7/1 -> Product_89b52/1
  State_psi_d_SG_D_1_fa460/1 -> Add_e7ea3/2
  Constant_x_dd_3736a/1 -> Subtract_b850d/1
  Constant_x_l_f444c/1 -> Subtract_1b8e7/2
  Constant_x_dd_c7d7e/1 -> Subtract_d68dd/1
  Subtract_21993/1 -> Product_a7042/2
  Constant_x_l_e512f/1 -> Subtract_b850d/2
  Divide_91c72/1 -> Subtract_aa658/2
  Constant_x_ddd_b9df0/1 -> Subtract_d68dd/2
  Constant_x_ddd_23f75/1 -> Subtract_21993/1
  Constant_x_l_8dddb/1 -> Subtract_21993/2
  Add_85150/1 -> Add_8d5e1/1
  Product_46e69/1 -> Divide_b306c/1
  Divide_50057/1 -> Add_8d5e1/2
  Subtract_b850d/1 -> Divide_b306c/2
  State_psi_fd_SG_D_1_43baf/1 -> Product_a7042/1
  Constant_x_dd_c88ae/1 -> Subtract_aa06c/1
  Constant_x_l_14475/1 -> Subtract_aa06c/2
  Constant_x_ddd_7d76a/1 -> Divide_50057/2
  Subtract_aa658/1 -> Product_89b52/2
  Divide_b306c/1 -> Add_e7ea3/1
  Product_a7042/1 -> Divide_91c72/1
  Subtract_aa06c/1 -> Divide_91c72/2
  Product_89b52/1 -> Divide_50057/1
  Constant_x_dd_aeb06/1 -> Subtract_1b8e7/1
  Add_e7ea3/1 -> Subtract_aa658/1
  Constant_-1_96109/1 -> Product_f0574/1
  State_psi_1d_SG_D_1_9b7db/1 -> Product_f0574/2
  Product_f0574/1 -> Add_85150/1
  State_psi_fd_SG_D_1_cc7fa/1 -> Add_85150/2
  Add_8d5e1/1 -> Divide_9ad1a/1
  Constant_T_ddd_e98c2/1 -> Divide_9ad1a/2
  Divide_9ad1a/1 -> Blockout_d_psi_1d_SG_D_1_2ff74/1

== system case2/SG_D_1/d_psi_d_SG_D_1_block ==
  note: d_psi_d_SG_D_1 in case2
      | $2\,\pi \,f_{0}\,\left(v_{d,\mathrm{SG},D,1}\,\sin\left(\theta _{\mathrm{SG},D,1}\right)-v_{q,\mathrm{SG},D,1}\,\cos\left(\theta _{\mathrm{SG},D,1}\right)+\frac{R_{a}\,\left(\frac{\psi _{\mathrm{1d},\mathrm{SG},D,1}\,\left(x_{\mathrm{dd}}-x_{\mathrm{ddd}}\right)}{x_{\mathrm{dd}}-x_{l}}-\psi _{d,\mathrm{SG},D,1}+\frac{\psi _{\mathrm{fd},\mathrm{SG},D,1}\,\left(x_{\mathrm{ddd}}-x_{l}\right)}{x_{\mathrm{dd}}-x_{l}}\right)}{x_{\mathrm{ddd}}}+\frac{\psi _{q,\mathrm{SG},D,1}\,w_{\mathrm{SG},D,1}}{2\,f_{0}\,\pi }\right)$
      | Automatically generated on 2025-10-31 18:52:46 .
  State_psi_1d_SG_D_1_71504 : Inport
  State_psi_d_SG_D_1_7243c : Inport  Port=2
  State_psi_fd_SG_D_1_71b08 : Inport  Port=3
  Input_v_d_SG_D_1_8f44e : Inport  Port=4
  State_theta_SG_D_1_4b996 : Inport  Port=5
  Input_v_q_SG_D_1_cfec8 : Inport  Port=6
  State_theta_SG_D_1_e6cd3 : Inport  Port=7
  State_psi_q_SG_D_1_21678 : Inport  Port=8
  State_w_SG_D_1_ca1da : Inport  Port=9
  Add_0140d : Sum
  Add_28ede : Sum
  Constant_-1_ad797 : Constant  Value=-1
  Constant_-2.0_e5efa : Constant  Value=-2.0
  Constant_2.0_9505d : Constant  Value=2.0
  Constant_R_a_27517 : Constant  Value=R_a
  Constant_f0_125a9 : Constant  Value=f0
  Constant_f0_18dfc : Constant  Value=f0
  Constant_pi_111c9 : Constant  Value=pi
  Constant_pi_900ba : Constant  Value=pi
  Constant_x_dd_726cc : Constant  Value=x_dd
  Constant_x_dd_c91d6 : Constant  Value=x_dd
  Constant_x_dd_ca9cf : Constant  Value=x_dd
  Constant_x_ddd_4e55d : Constant  Value=x_ddd
  Constant_x_ddd_904d1 : Constant  Value=x_ddd
  Constant_x_ddd_d1278 : Constant  Value=x_ddd
  Constant_x_l_29bf5 : Constant  Value=x_l
  Constant_x_l_392ee : Constant  Value=x_l
  Constant_x_l_3f6df : Constant  Value=x_l
  Divide_1eb30 : Product  Inputs=*/
  Divide_2818b : Product  Inputs=*/
  Divide_6873a : Product  Inputs=*/
  Divide_da29e : Product  Inputs=*/
  MathFunc_cos_9103d : Trigonometry  Operator=cos
  MathFunc_sin_1ef12 : Trigonometry
  Product_01085 : Product
  Product_05291 : Product
  Product_0bbc8 : Product
  Product_2616a : Product
  Product_28904 : Product
  Product_45ee9 : Product
  Product_addf5 : Product
  Product_bc770 : Product
  Product_ce40c : Product
  Product_d1068 : Product
  Product_e9ccd : Product
  Product_f5657 : Product
  Subtract_0eb20 : Sum  Inputs=+-
  Subtract_26380 : Sum  Inputs=+-
  Subtract_56469 : Sum  Inputs=+-
  Subtract_ab1c0 : Sum  Inputs=+-
  Subtract_b1aaf : Sum  Inputs=+-
  Subtract_f8034 : Sum  Inputs=+-
  Subtract_fa564 : Sum  Inputs=+-
  Blockout_d_psi_d_SG_D_1_ed5ed : Outport
  wires:
  Add_0140d/1 -> Subtract_b1aaf/1
  Product_28904/1 -> Divide_1eb30/1
  Subtract_f8034/1 -> Product_28904/2
  Divide_1eb30/1 -> Add_0140d/1
  Product_2616a/1 -> Product_28904/1
  Constant_x_ddd_d1278/1 -> Subtract_f8034/2
  Constant_x_dd_c91d6/1 -> Subtract_f8034/1
  State_psi_1d_SG_D_1_71504/1 -> Product_2616a/2
  Constant_-1_ad797/1 -> Product_2616a/1
  Product_45ee9/1 -> Divide_da29e/1
  Constant_x_l_29bf5/1 -> Subtract_ab1c0/2
  State_psi_d_SG_D_1_7243c/1 -> Add_0140d/2
  Constant_x_dd_ca9cf/1 -> Subtract_ab1c0/1
  Constant_x_ddd_4e55d/1 -> Subtract_0eb20/1
  Constant_x_l_392ee/1 -> Subtract_0eb20/2
  Subtract_ab1c0/1 -> Divide_1eb30/2
  State_psi_fd_SG_D_1_71b08/1 -> Product_45ee9/1
  Constant_x_ddd_904d1/1 -> Divide_2818b/2
  Subtract_0eb20/1 -> Product_45ee9/2
  Product_0bbc8/1 -> Subtract_fa564/2
  Constant_x_dd_726cc/1 -> Subtract_56469/1
  Constant_x_l_3f6df/1 -> Subtract_56469/2
  Subtract_56469/1 -> Divide_da29e/2
  Divide_da29e/1 -> Subtract_b1aaf/2
  Constant_R_a_27517/1 -> Product_d1068/1
  Subtract_b1aaf/1 -> Product_d1068/2
  MathFunc_cos_9103d/1 -> Product_01085/2
  State_theta_SG_D_1_4b996/1 -> MathFunc_sin_1ef12/1
  Divide_2818b/1 -> Subtract_fa564/1
  Product_d1068/1 -> Divide_2818b/1
  MathFunc_sin_1ef12/1 -> Product_0bbc8/2
  Input_v_d_SG_D_1_8f44e/1 -> Product_0bbc8/1
  Product_e9ccd/1 -> Blockout_d_psi_d_SG_D_1_ed5ed/1
  Product_ce40c/1 -> Product_e9ccd/1
  Product_bc770/1 -> Product_ce40c/1
  State_theta_SG_D_1_e6cd3/1 -> MathFunc_cos_9103d/1
  Constant_2.0_9505d/1 -> Product_f5657/1
  Constant_pi_111c9/1 -> Product_f5657/2
  Input_v_q_SG_D_1_cfec8/1 -> Product_01085/1
  Constant_f0_18dfc/1 -> Product_ce40c/2
  State_psi_q_SG_D_1_21678/1 -> Product_addf5/1
  State_w_SG_D_1_ca1da/1 -> Product_addf5/2
  Product_f5657/1 -> Product_05291/1
  Constant_pi_900ba/1 -> Product_bc770/2
  Constant_f0_125a9/1 -> Product_05291/2
  Constant_-2.0_e5efa/1 -> Product_bc770/1
  Add_28ede/1 -> Subtract_26380/1
  Subtract_fa564/1 -> Add_28ede/1
  Product_01085/1 -> Add_28ede/2
  Product_addf5/1 -> Divide_6873a/1
  Product_05291/1 -> Divide_6873a/2
  Divide_6873a/1 -> Subtract_26380/2
  Subtract_26380/1 -> Product_e9ccd/2

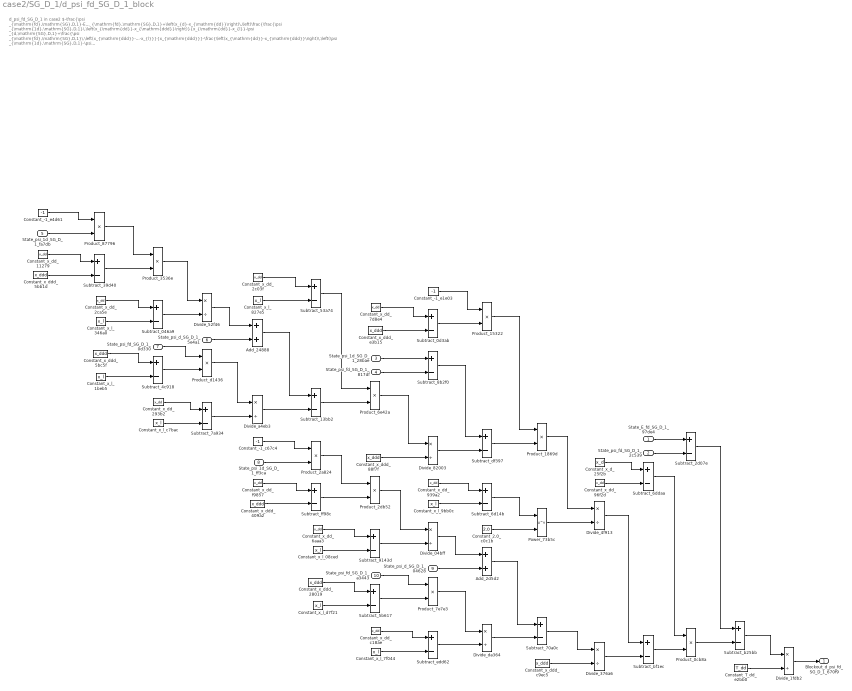
== system case2/SG_D_1/d_psi_fd_SG_D_1_block ==
  note: d_psi_fd_SG_D_1 in case2
      | $-\frac{\psi _{\mathrm{fd},\mathrm{SG},D,1}-E_{\mathrm{fd},\mathrm{SG},D,1}+\left(x_{d}-x_{\mathrm{dd}}\right)\,\left(\frac{\frac{\psi _{\mathrm{1d},\mathrm{SG},D,1}\,\left(x_{\mathrm{dd}}-x_{\mathrm{ddd}}\right)}{x_{\mathrm{dd}}-x_{l}}-\psi _{d,\mathrm{SG},D,1}+\frac{\psi _{\mathrm{fd},\mathrm{SG},D,1}\,\left(x_{\mathrm{ddd}}-x_{l}\right)}{x_{\mathrm{dd}}-x_{l}}}{x_{\mathrm{ddd}}}-\frac{\left(x_{\mathrm{dd}}-x_{\mathrm{ddd}}\right)\,\left(\psi _{\mathrm{1d},\mathrm{SG},D,1}-\psi _{\mathrm{fd},\mathrm{SG},D,1}+\frac{\left(x_{\mathrm{dd}}-x_{l}\right)\,\left(\frac{\psi _{\mathrm{1d},\mathrm{SG},D,1}\,\left(x_{\mathrm{dd}}-x_{\mathrm{ddd}}\right)}{x_{\mathrm{dd}}-x_{l}}-\psi _{d,\mathrm{SG},D,1}+\frac{\psi _{\mathrm{fd},\mathrm{SG},D,1}\,\left(x_{\mathrm{ddd}}-x_{l}\right)}{x_{\mathrm{dd}}-x_{l}}\right)}{x_{\mathrm{ddd}}}\right)}{{\left(x_{\mathrm{dd}}-x_{l}\right)}^2}\right)}{T_{\mathrm{dd}}}$
      | Automatically generated on 2025-10-31 18:53:10 .
  State_E_fd_SG_D_1_97de4 : Inport
  State_psi_fd_SG_D_1_2c539 : Inport  Port=2
  State_psi_1d_SG_D_1_28bae : Inport  Port=3
  State_psi_fd_SG_D_1_817df : Inport  Port=4
  State_psi_1d_SG_D_1_fa7db : Inport  Port=5
  State_psi_d_SG_D_1_5e4a1 : Inport  Port=6
  State_psi_fd_SG_D_1_0d330 : Inport  Port=7
  State_psi_1d_SG_D_1_ff3ca : Inport  Port=8
  State_psi_d_SG_D_1_04628 : Inport  Port=9
  State_psi_fd_SG_D_1_a3443 : Inport  Port=10
  Add_24888 : Sum
  Add_2d5d2 : Sum
  Constant_-1_c67c4 : Constant  Value=-1
  Constant_-1_e1e03 : Constant  Value=-1
  Constant_-1_e4d61 : Constant  Value=-1
  Constant_2.0_c0c1b : Constant  Value=2.0
  Constant_T_dd_e2bb0 : Constant  Value=T_dd
  Constant_x_d_25f2b : Constant  Value=x_d
  Constant_x_dd_11279 : Constant  Value=x_dd
  Constant_x_dd_293b2 : Constant  Value=x_dd
  Constant_x_dd_2c03f : Constant  Value=x_dd
  Constant_x_dd_2ca5e : Constant  Value=x_dd
  Constant_x_dd_6aaa3 : Constant  Value=x_dd
  Constant_x_dd_7d8e4 : Constant  Value=x_dd
  Constant_x_dd_939a2 : Constant  Value=x_dd
  Constant_x_dd_96f2d : Constant  Value=x_dd
  Constant_x_dd_c18ae : Constant  Value=x_dd
  Constant_x_dd_f9857 : Constant  Value=x_dd
  Constant_x_ddd_28019 : Constant  Value=x_ddd
  Constant_x_ddd_409a2 : Constant  Value=x_ddd
  Constant_x_ddd_5bb1d : Constant  Value=x_ddd
  Constant_x_ddd_5bc5f : Constant  Value=x_ddd
  Constant_x_ddd_88f7f : Constant  Value=x_ddd
  Constant_x_ddd_c9ec5 : Constant  Value=x_ddd
  Constant_x_ddd_e3b15 : Constant  Value=x_ddd
  Constant_x_l_08ced : Constant  Value=x_l
  Constant_x_l_1beb5 : Constant  Value=x_l
  Constant_x_l_346a0 : Constant  Value=x_l
  Constant_x_l_7f044 : Constant  Value=x_l
  Constant_x_l_827e5 : Constant  Value=x_l
  Constant_x_l_9bb0c : Constant  Value=x_l
  Constant_x_l_c7bac : Constant  Value=x_l
  Constant_x_l_d7f21 : Constant  Value=x_l
  Divide_04bff : Product  Inputs=*/
  Divide_1fdb2 : Product  Inputs=*/
  Divide_376a6 : Product  Inputs=*/
  Divide_4f913 : Product  Inputs=*/
  Divide_52f46 : Product  Inputs=*/
  Divide_82003 : Product  Inputs=*/
  Divide_a4eb3 : Product  Inputs=*/
  Divide_da364 : Product  Inputs=*/
  Power_73b5c : Math  Operator=pow
  Product_0cb8a : Product
  Product_15322 : Product
  Product_1869d : Product
  Product_2a824 : Product
  Product_2db52 : Product
  Product_3536e : Product
  Product_6e42a : Product
  Product_7e7e3 : Product
  Product_87796 : Product
  Product_d1436 : Product
  Subtract_046a9 : Sum  Inputs=+-
  Subtract_0d3ab : Sum  Inputs=+-
  Subtract_13bb2 : Sum  Inputs=+-
  Subtract_2d07e : Sum  Inputs=+-
  Subtract_39d40 : Sum  Inputs=+-
  Subtract_4c918 : Sum  Inputs=+-
  Subtract_53a74 : Sum  Inputs=+-
  Subtract_5b617 : Sum  Inputs=+-
  Subtract_6d14b : Sum  Inputs=+-
  Subtract_6ddaa : Sum  Inputs=+-
  Subtract_70a0c : Sum  Inputs=+-
  Subtract_7a934 : Sum  Inputs=+-
  Subtract_8b2f0 : Sum  Inputs=+-
  Subtract_9143d : Sum  Inputs=+-
  Subtract_b25bb : Sum  Inputs=+-
  Subtract_bf1ec : Sum  Inputs=+-
  Subtract_df397 : Sum  Inputs=+-
  Subtract_edd62 : Sum  Inputs=+-
  Subtract_ff98c : Sum  Inputs=+-
  Blockout_d_psi_fd_SG_D_1_670f9 : Outport
  wires:
  State_psi_d_SG_D_1_5e4a1/1 -> Add_24888/2
  Constant_x_dd_2ca5e/1 -> Subtract_046a9/1
  Product_3536e/1 -> Divide_52f46/1
  Subtract_39d40/1 -> Product_3536e/2
  Subtract_13bb2/1 -> Product_6e42a/2
  Product_87796/1 -> Product_3536e/1
  Constant_x_dd_11279/1 -> Subtract_39d40/1
  Constant_x_l_827e5/1 -> Subtract_53a74/2
  Constant_-1_e4d61/1 -> Product_87796/1
  Subtract_53a74/1 -> Product_6e42a/1
  Constant_x_l_346a0/1 -> Subtract_046a9/2
  Constant_x_ddd_5bb1d/1 -> Subtract_39d40/2
  State_psi_1d_SG_D_1_fa7db/1 -> Product_87796/2
  Constant_x_ddd_5bc5f/1 -> Subtract_4c918/1
  Constant_x_l_1beb5/1 -> Subtract_4c918/2
  State_E_fd_SG_D_1_97de4/1 -> Subtract_2d07e/1
  Divide_52f46/1 -> Add_24888/1
  Subtract_046a9/1 -> Divide_52f46/2
  State_psi_fd_SG_D_1_0d330/1 -> Product_d1436/1
  Constant_x_ddd_88f7f/1 -> Divide_82003/2
  Subtract_4c918/1 -> Product_d1436/2
  Constant_x_dd_293b2/1 -> Subtract_7a934/1
  Constant_x_dd_939a2/1 -> Subtract_6d14b/1
  State_psi_fd_SG_D_1_2c539/1 -> Subtract_2d07e/2
  Constant_x_l_c7bac/1 -> Subtract_7a934/2
  Product_d1436/1 -> Divide_a4eb3/1
  Constant_-1_e1e03/1 -> Product_15322/1
  Subtract_7a934/1 -> Divide_a4eb3/2
  Constant_x_dd_2c03f/1 -> Subtract_53a74/1
  Add_24888/1 -> Subtract_13bb2/1
  Constant_x_l_9bb0c/1 -> Subtract_6d14b/2
  Divide_a4eb3/1 -> Subtract_13bb2/2
  Divide_4f913/1 -> Subtract_bf1ec/1
  Constant_-1_c67c4/1 -> Product_2a824/1
  State_psi_1d_SG_D_1_ff3ca/1 -> Product_2a824/2
  Constant_x_dd_f9857/1 -> Subtract_ff98c/1
  Subtract_0d3ab/1 -> Product_15322/2
  Constant_x_ddd_409a2/1 -> Subtract_ff98c/2
  Product_2a824/1 -> Product_2db52/1
  Constant_2.0_c0c1b/1 -> Power_73b5c/2
  Product_2db52/1 -> Divide_04bff/1
  Subtract_bf1ec/1 -> Product_0cb8a/2
  Subtract_ff98c/1 -> Product_2db52/2
  State_psi_d_SG_D_1_04628/1 -> Add_2d5d2/2
  Constant_x_dd_6aaa3/1 -> Subtract_9143d/1
  Constant_x_l_08ced/1 -> Subtract_9143d/2
  Constant_x_dd_7d8e4/1 -> Subtract_0d3ab/1
  Divide_82003/1 -> Subtract_df397/2
  Constant_x_ddd_28019/1 -> Subtract_5b617/1
  Constant_x_ddd_e3b15/1 -> Subtract_0d3ab/2
  Constant_x_l_d7f21/1 -> Subtract_5b617/2
  Subtract_5b617/1 -> Product_7e7e3/2
  State_psi_1d_SG_D_1_28bae/1 -> Subtract_8b2f0/1
  Product_7e7e3/1 -> Divide_da364/1
  State_psi_fd_SG_D_1_817df/1 -> Subtract_8b2f0/2
  State_psi_fd_SG_D_1_a3443/1 -> Product_7e7e3/1
  Product_6e42a/1 -> Divide_82003/1
  Divide_04bff/1 -> Add_2d5d2/1
  Subtract_9143d/1 -> Divide_04bff/2
  Constant_x_dd_c18ae/1 -> Subtract_edd62/1
  Constant_x_l_7f044/1 -> Subtract_edd62/2
  Divide_da364/1 -> Subtract_70a0c/2
  Subtract_8b2f0/1 -> Subtract_df397/1
  Subtract_edd62/1 -> Divide_da364/2
  Subtract_df397/1 -> Product_1869d/2
  Product_15322/1 -> Product_1869d/1
  Subtract_6d14b/1 -> Power_73b5c/1
  Add_2d5d2/1 -> Subtract_70a0c/1
  Product_1869d/1 -> Divide_4f913/1
  Power_73b5c/1 -> Divide_4f913/2
  Subtract_70a0c/1 -> Divide_376a6/1
  Constant_x_ddd_c9ec5/1 -> Divide_376a6/2
  Constant_x_d_25f2b/1 -> Subtract_6ddaa/1
  Constant_x_dd_96f2d/1 -> Subtract_6ddaa/2
  Divide_376a6/1 -> Subtract_bf1ec/2
  Subtract_6ddaa/1 -> Product_0cb8a/1
  Subtract_2d07e/1 -> Subtract_b25bb/1
  Product_0cb8a/1 -> Subtract_b25bb/2
  Subtract_b25bb/1 -> Divide_1fdb2/1
  Constant_T_dd_e2bb0/1 -> Divide_1fdb2/2
  Divide_1fdb2/1 -> Blockout_d_psi_fd_SG_D_1_670f9/1

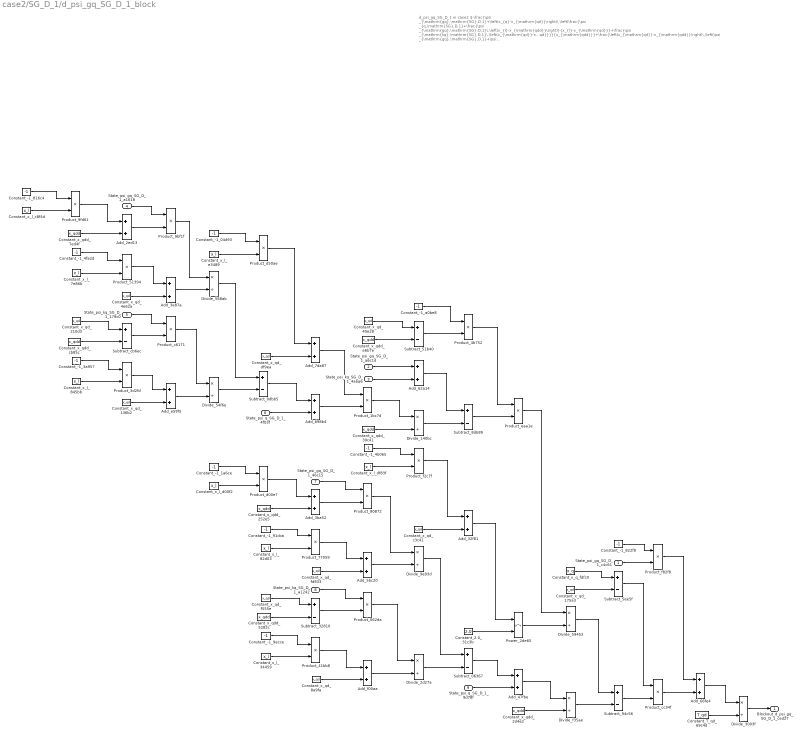
== system case2/SG_D_1/d_psi_gq_SG_D_1_block ==
  note: d_psi_gq_SG_D_1 in case2
      | $-\frac{\psi _{\mathrm{gq},\mathrm{SG},D,1}+\left(x_{q}-x_{\mathrm{qd}}\right)\,\left(\frac{\psi _{q,\mathrm{SG},D,1}+\frac{\psi _{\mathrm{gq},\mathrm{SG},D,1}\,\left(x_{l}-x_{\mathrm{qdd}}\right)}{x_{l}-x_{\mathrm{qd}}}+\frac{\psi _{\mathrm{kq},\mathrm{SG},D,1}\,\left(x_{\mathrm{qd}}-x_{\mathrm{qdd}}\right)}{x_{l}-x_{\mathrm{qd}}}}{x_{\mathrm{qdd}}}+\frac{\left(x_{\mathrm{qd}}-x_{\mathrm{qdd}}\right)\,\left(\psi _{\mathrm{gq},\mathrm{SG},D,1}+\psi _{\mathrm{kq},\mathrm{SG},D,1}+\frac{\left(x_{l}-x_{\mathrm{qd}}\right)\,\left(\psi _{q,\mathrm{SG},D,1}+\frac{\psi _{\mathrm{gq},\mathrm{SG},D,1}\,\left(x_{l}-x_{\mathrm{qdd}}\right)}{x_{l}-x_{\mathrm{qd}}}+\frac{\psi _{\mathrm{kq},\mathrm{SG},D,1}\,\left(x_{\mathrm{qd}}-x_{\mathrm{qdd}}\right)}{x_{l}-x_{\mathrm{qd}}}\right)}{x_{\mathrm{qdd}}}\right)}{{\left(x_{l}-x_{\mathrm{qd}}\right)}^2}\right)}{T_{\mathrm{qd}}}$
      | Automatically generated on 2025-10-31 18:53:19 .
  State_psi_gq_SG_D_1_c4c61 : Inport
  State_psi_gq_SG_D_1_a6c1d : Inport  Port=2
  State_psi_kq_SG_D_1_4aba6 : Inport  Port=3
  State_psi_gq_SG_D_1_a1618 : Inport  Port=4
  State_psi_kq_SG_D_1_179c0 : Inport  Port=5
  State_psi_q_SG_D_1_4f03f : Inport  Port=6
  State_psi_gq_SG_D_1_46c15 : Inport  Port=7
  State_psi_kq_SG_D_1_a1242 : Inport  Port=8
  State_psi_q_SG_D_1_9d78f : Inport  Port=9
  Add_2ed13 : Sum
  Add_32f81 : Sum
  Add_3ba52 : Sum
  Add_3e87a : Sum
  Add_47fbe : Sum
  Add_5bc20 : Sum
  Add_62a14 : Sum
  Add_66fe4 : Sum
  Add_698b4 : Sum
  Add_7da87 : Sum
  Add_e59f5 : Sum
  Add_f00aa : Sum
  Constant_-1_04d93 : Constant  Value=-1
  Constant_-1_1a6ce : Constant  Value=-1
  Constant_-1_3a957 : Constant  Value=-1
  Constant_-1_4b065 : Constant  Value=-1
  Constant_-1_4fa2d : Constant  Value=-1
  Constant_-1_816c4 : Constant  Value=-1
  Constant_-1_822f8 : Constant  Value=-1
  Constant_-1_91cba : Constant  Value=-1
  Constant_-1_9ecce : Constant  Value=-1
  Constant_-1_a0be8 : Constant  Value=-1
  Constant_2.0_31c3b : Constant  Value=2.0
  Constant_T_qd_69c4d : Constant  Value=T_qd
  Constant_x_l_34459 : Constant  Value=x_l
  Constant_x_l_7e86b : Constant  Value=x_l
  Constant_x_l_82d03 : Constant  Value=x_l
  Constant_x_l_845bb : Constant  Value=x_l
  Constant_x_l_c8f4d : Constant  Value=x_l
  Constant_x_l_d00f2 : Constant  Value=x_l
  Constant_x_l_df83f : Constant  Value=x_l
  Constant_x_l_e3489 : Constant  Value=x_l
  Constant_x_q_fdfc0 : Constant  Value=x_q
  Constant_x_qd_136b2 : Constant  Value=x_qd
  Constant_x_qd_175a3 : Constant  Value=x_qd
  Constant_x_qd_210d3 : Constant  Value=x_qd
  Constant_x_qd_40e28 : Constant  Value=x_qd
  Constant_x_qd_4e62a : Constant  Value=x_qd
  Constant_x_qd_8a9fa : Constant  Value=x_qd
  Constant_x_qd_c3c41 : Constant  Value=x_qd
  Constant_x_qd_df9ea : Constant  Value=x_qd
  Constant_x_qd_f555e : Constant  Value=x_qd
  Constant_x_qd_fd833 : Constant  Value=x_qd
  Constant_x_qdd_252e5 : Constant  Value=x_qdd
  Constant_x_qdd_2d4e2 : Constant  Value=x_qdd
  Constant_x_qdd_39c41 : Constant  Value=x_qdd
  Constant_x_qdd_5282c : Constant  Value=x_qdd
  Constant_x_qdd_7ed4f : Constant  Value=x_qdd
  Constant_x_qdd_cb85c : Constant  Value=x_qdd
  Constant_x_qdd_e6b7e : Constant  Value=x_qdd
  Divide_140bc : Product  Inputs=*/
  Divide_2d27a : Product  Inputs=*/
  Divide_3003f : Product  Inputs=*/
  Divide_54f6e : Product  Inputs=*/
  Divide_568ab : Product  Inputs=*/
  Divide_59453 : Product  Inputs=*/
  Divide_9e93d : Product  Inputs=*/
  Divide_f35ae : Product  Inputs=*/
  Power_2de65 : Math  Operator=pow
  Product_062da : Product
  Product_1bc7d : Product
  Product_3d2fd : Product
  Product_41bb8 : Product
  Product_4b752 : Product
  Product_51394 : Product
  Product_77059 : Product
  Product_80872 : Product
  Product_9bf1f : Product
  Product_9fd61 : Product
  Product_c6171 : Product
  Product_cc34f : Product
  Product_d00e7 : Product
  Product_d50ae : Product
  Product_eaa1e : Product
  Product_f2c7f : Product
  Product_f82f8 : Product
  Subtract_06367 : Sum  Inputs=+-
  Subtract_0dbb5 : Sum  Inputs=+-
  Subtract_32810 : Sum  Inputs=+-
  Subtract_51b40 : Sum  Inputs=+-
  Subtract_5ee5f : Sum  Inputs=+-
  Subtract_8db89 : Sum  Inputs=+-
  Subtract_94c56 : Sum  Inputs=+-
  Subtract_cb6ec : Sum  Inputs=+-
  Blockout_d_psi_gq_SG_D_1_ced27 : Outport
  wires:
  State_psi_gq_SG_D_1_a1618/1 -> Product_9bf1f/1
  Constant_-1_4fa2d/1 -> Product_51394/1
  Divide_568ab/1 -> Subtract_0dbb5/1
  Add_3e87a/1 -> Divide_568ab/2
  Product_9fd61/1 -> Add_2ed13/1
  Constant_x_qd_df9ea/1 -> Add_7da87/2
  Constant_-1_816c4/1 -> Product_9fd61/1
  Constant_x_qdd_7ed4f/1 -> Add_2ed13/2
  Constant_x_l_7e86b/1 -> Product_51394/2
  Constant_x_l_c8f4d/1 -> Product_9fd61/2
  Constant_-1_3a957/1 -> Product_3d2fd/1
  Constant_x_qd_210d3/1 -> Subtract_cb6ec/1
  Constant_x_qdd_39c41/1 -> Divide_140bc/2
  Constant_x_l_845bb/1 -> Product_3d2fd/2
  Constant_x_qdd_cb85c/1 -> Subtract_cb6ec/2
  Subtract_0dbb5/1 -> Add_698b4/1
  Add_2ed13/1 -> Product_9bf1f/2
  Product_9bf1f/1 -> Divide_568ab/1
  Product_51394/1 -> Add_3e87a/1
  Constant_x_qd_4e62a/1 -> Add_3e87a/2
  State_psi_kq_SG_D_1_179c0/1 -> Product_c6171/1
  Product_3d2fd/1 -> Add_e59f5/1
  Subtract_cb6ec/1 -> Product_c6171/2
  Constant_x_qd_136b2/1 -> Add_e59f5/2
  Product_c6171/1 -> Divide_54f6e/1
  Add_e59f5/1 -> Divide_54f6e/2
  Constant_-1_a0be8/1 -> Product_4b752/1
  Constant_-1_04d93/1 -> Product_d50ae/1
  Add_5bc20/1 -> Divide_9e93d/2
  Product_41bb8/1 -> Add_f00aa/1
  Subtract_32810/1 -> Product_062da/2
  Constant_x_l_e3489/1 -> Product_d50ae/2
  Divide_54f6e/1 -> Subtract_0dbb5/2
  Subtract_5ee5f/1 -> Product_cc34f/1
  Constant_-1_4b065/1 -> Product_f2c7f/1
  Constant_-1_1a6ce/1 -> Product_d00e7/1
  Constant_x_l_df83f/1 -> Product_f2c7f/2
  Constant_x_l_d00f2/1 -> Product_d00e7/2
  Constant_x_qd_fd833/1 -> Add_5bc20/2
  Product_d50ae/1 -> Add_7da87/1
  State_psi_q_SG_D_1_4f03f/1 -> Add_698b4/2
  Product_d00e7/1 -> Add_3ba52/1
  Constant_x_qdd_252e5/1 -> Add_3ba52/2
  Constant_-1_91cba/1 -> Product_77059/1
  Constant_x_qd_8a9fa/1 -> Add_f00aa/2
  Add_7da87/1 -> Product_1bc7d/1
  Constant_x_l_82d03/1 -> Product_77059/2
  Constant_-1_9ecce/1 -> Product_41bb8/1
  Constant_x_qd_f555e/1 -> Subtract_32810/1
  Product_1bc7d/1 -> Divide_140bc/1
  Constant_x_l_34459/1 -> Product_41bb8/2
  Divide_59453/1 -> Subtract_94c56/1
  Constant_x_qdd_5282c/1 -> Subtract_32810/2
  Add_698b4/1 -> Product_1bc7d/2
  State_psi_gq_SG_D_1_46c15/1 -> Product_80872/1
  Add_3ba52/1 -> Product_80872/2
  Product_77059/1 -> Add_5bc20/1
  State_psi_kq_SG_D_1_a1242/1 -> Product_062da/1
  Add_f00aa/1 -> Divide_2d27a/2
  State_psi_gq_SG_D_1_a6c1d/1 -> Add_62a14/1
  Constant_x_qd_40e28/1 -> Subtract_51b40/1
  Constant_x_qdd_e6b7e/1 -> Subtract_51b40/2
  Product_062da/1 -> Divide_2d27a/1
  State_psi_kq_SG_D_1_4aba6/1 -> Add_62a14/2
  Product_80872/1 -> Divide_9e93d/1
  Subtract_51b40/1 -> Product_4b752/2
  Add_62a14/1 -> Subtract_8db89/1
  Divide_140bc/1 -> Subtract_8db89/2
  Product_f2c7f/1 -> Add_32f81/1
  Constant_x_qd_c3c41/1 -> Add_32f81/2
  Divide_9e93d/1 -> Subtract_06367/1
  Divide_2d27a/1 -> Subtract_06367/2
  Product_4b752/1 -> Product_eaa1e/1
  Subtract_8db89/1 -> Product_eaa1e/2
  Add_32f81/1 -> Power_2de65/1
  Constant_2.0_31c3b/1 -> Power_2de65/2
  Subtract_06367/1 -> Add_47fbe/1
  State_psi_q_SG_D_1_9d78f/1 -> Add_47fbe/2
  Product_eaa1e/1 -> Divide_59453/1
  Power_2de65/1 -> Divide_59453/2
  Add_47fbe/1 -> Divide_f35ae/1
  Constant_x_qdd_2d4e2/1 -> Divide_f35ae/2
  Constant_x_q_fdfc0/1 -> Subtract_5ee5f/1
  Constant_x_qd_175a3/1 -> Subtract_5ee5f/2
  Divide_f35ae/1 -> Subtract_94c56/2
  Constant_-1_822f8/1 -> Product_f82f8/1
  State_psi_gq_SG_D_1_c4c61/1 -> Product_f82f8/2
  Subtract_94c56/1 -> Product_cc34f/2
  Product_f82f8/1 -> Add_66fe4/1
  Product_cc34f/1 -> Add_66fe4/2
  Add_66fe4/1 -> Divide_3003f/1
  Constant_T_qd_69c4d/1 -> Divide_3003f/2
  Divide_3003f/1 -> Blockout_d_psi_gq_SG_D_1_ced27/1
